simulink model "rossler_attractor"  (R2024a)
settings: Solver=VariableStepAuto  StartTime=0.0  StopTime=100.0  RelTol=1e-3
settings Model: PacingRate=0.990000  Creator=konga  LastModifiedBy=konga
settings DataIOCC: SaveFormat=Array

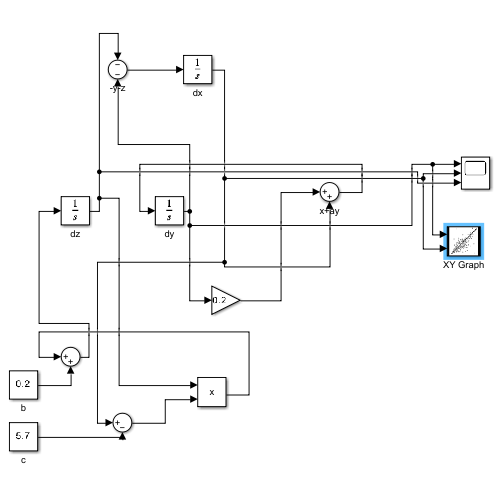
[thumbnail: Simulink's stored preview of the top-level diagram]
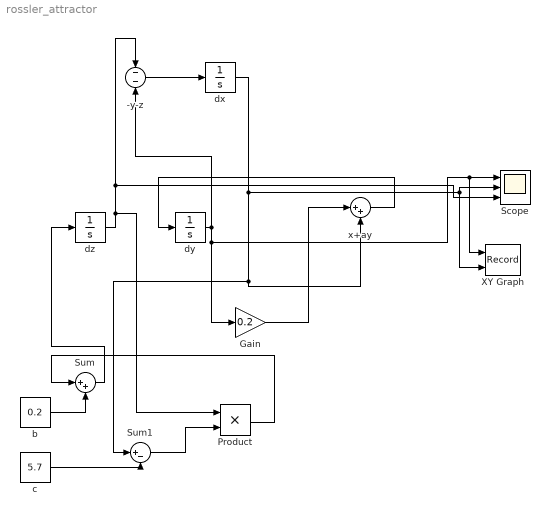
== system rossler_attractor ==
  -y-z : Sum  Inputs=--
  Gain : Gain  Gain=0.2
  Product : Product
  Scope : Scope  NumInputPorts=3
  Sum : Sum  Inputs=|++
  Sum1 : Sum  Inputs=|+-
  XY Graph : Record  VariableName=recordXY  Filename=C:\Users\konga\Desktop\test.mldatx  RecordToWorkspace=on  RecordToFile=on  FileSettingsInternal="{\"entries\":[{\"content\":{\"excelSettings\":{\"content\":{},\"type\":\"Streamout.ExcelSettings\"}},\"type\":\"Streamout.FileSettingStorage\",\"uuid\":\"\"}],\"packageUris\":[\"http:\\/\\/schema.mathworks.com\\/mf0\\/streamout_blocks\\/R2020a\"],\"version\":\"1.0\"}"  Layout=[1 1]  SignalsInternal="{\"entries\":[{\"content\":{\"signals\":[{\"content\":{\"blockPath\":[],\"dimensions\":[1],\"domain\":\"\",\"lineColor\":\"#a2142f\",\"plots\":[ 1 ],\"port\":1,\"sid\":[\"\"],\"signalID\":1,\"signalName\":\"dy\"},\"type\":\"RecordBlkView.Signal\",\"uuid\":\"\"},{\"content\":{\"blockPath\":[],\"dimensions\":[1],\"domain\":\"\",\"lineColor\":\"#139fff\",\"plots\":[ 1 ],\"port\":2,\"sid\":[\"\"],\"signalID\":2,\"signalName\":\"dx\"},\"type\":\"RecordBlkView.Signal\",\"uuid\":\"\"}]},\"type\":\"RecordBlkView.InputSignals\",\"uuid\":\"\"}],\"packageUris\":[\"http:\\/\\/schema.mathworks.com\\/mf0\\/streamout_blocks\\/R2020a\"],\"version\":\"1.0\"}"  CompatibilityTag=XY
  b : Constant  Value=0.2
  c : Constant  Value=5.7
  dx : Integrator
  dy : Integrator
  dz : Integrator
  x+ay : Sum  Inputs=|++
  wires:
  dy/1 -> -y-z/2, XY Graph/1, Scope/1, Gain/1
  dz/1 -> Scope/3, -y-z/1, Product/1
  -y-z/1 -> dx/1
  dx/1 -> XY Graph/2, Scope/2, Sum1/1, x+ay/2
  Gain/1 -> x+ay/1
  x+ay/1 -> dy/1
  b/1 -> Sum/2
  c/1 -> Sum1/2
  Sum1/1 -> Product/2
  Product/1 -> Sum/1
  Sum/1 -> dz/1
